simulink model "DyskM"  (R2023b)
settings: Solver=ode4  StartTime=0.0  StopTime=7  FixedStep=0.001  RelTol=1e-3
undefined symbols (not defined in the file): A, A_plus, B, B_plus, C, C_plus, D_plus, h
settings Model: Creator=Andrzej  LastModifiedBy=roman
settings DataIOCC: ReturnWorkspaceOutputs=off

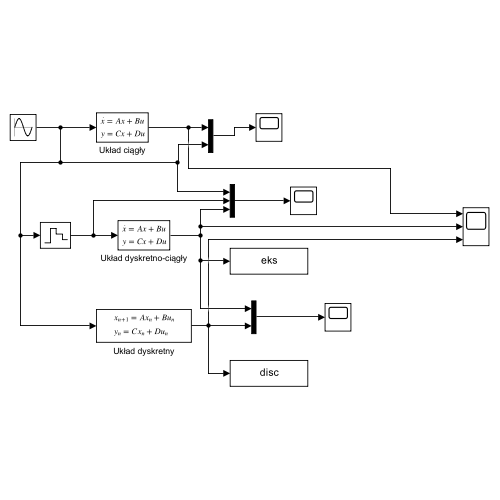
[thumbnail: Simulink's stored preview of the top-level diagram]
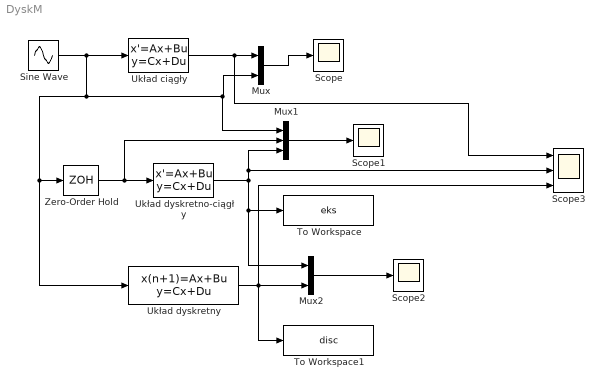
== system DyskM ==
  Mux : Mux  Inputs=2
  Mux1 : Mux  Inputs=3
  Mux2 : Mux  Inputs=2
  Scope : Scope
  Scope1 : Scope
  Scope2 : Scope
  Scope3 : Scope  NumInputPorts=3
  Sine Wave : Sin  Bias=1  SampleTime=0
  To Workspace : ToWorkspace  VariableName=eks  SaveFormat=Structure With Time  SampleTime=0.001
      settings: Save2DSignal=2-D array (concatenate along first dimension)
  To Workspace1 : ToWorkspace  VariableName=disc  SaveFormat=Structure With Time  SampleTime=0.001
      settings: Save2DSignal=2-D array (concatenate along first dimension)
  Układ ciągły : StateSpace  A=A  B=B  C=C  D=[0]  InitialCondition=[1; 0]
  Układ dyskretno-ciągły : StateSpace  A=A  B=B  C=C  D=[0]  InitialCondition=[1;0]
  Układ dyskretny : DiscreteStateSpace  A=A_plus(h)  B=double(B_plus)  C=C_plus  D=D_plus  InitialCondition=[1;0]  SampleTime=round(h,3)
  Zero-Order Hold : ZeroOrderHold  SampleTime=round(h, 3)
  wires:
  Sine Wave/1 -> Układ dyskretny/1, Zero-Order Hold/1, Mux1/1, Mux/2, Układ ciągły/1
  Układ ciągły/1 -> Scope3/1, Mux/1
  Mux/1 -> Scope/1
  Zero-Order Hold/1 -> Mux1/2, Układ dyskretno-ciągły/1
  Mux1/1 -> Scope1/1
  Układ dyskretno-ciągły/1 -> Mux1/3, Scope3/2, Mux2/1, To Workspace/1
  Mux2/1 -> Scope2/1
  Układ dyskretny/1 -> To Workspace1/1, Scope3/3, Mux2/2
